simulink model "Quadrotor_Model_Roll"  (R2016a)
settings: Solver=ode45  StartTime=0.0  StopTime=20  MinStep=1e-10  RelTol=1e-1
settings Model: Creator=SRQ  LastModifiedBy=SRQ

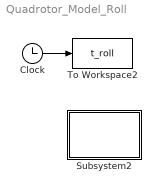
== system Quadrotor_Model_Roll ==
  Clock : Clock
  Subsystem2 : Subsystem
      mask Display: disp('翻滚通道');
  To Workspace2 : ToWorkspace  VariableName=t_roll  SampleTime=-1
  wires:
  Clock/1 -> To Workspace2/1

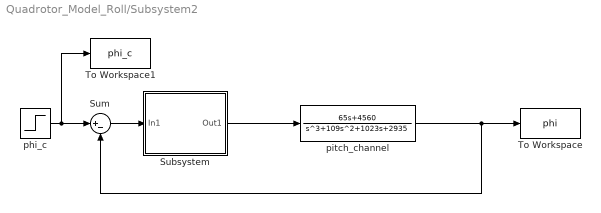
== system Quadrotor_Model_Roll/Subsystem2 ==
  Subsystem : Subsystem  mask{kp=2, ki=6, kd=0.1}
      mask Display: disp('PID');
  Sum : Sum  Inputs=|+-
  To Workspace : ToWorkspace  VariableName=phi  SampleTime=-1
  To Workspace1 : ToWorkspace  VariableName=phi_c  SampleTime=-1
  phi_c : Step  Time=0  SampleTime=0
  pitch_channel : TransferFcn  Numerator=[65 4560]  Denominator=[1 109 1023 2935]
  wires:
  phi_c/1 -> To Workspace1/1, Sum/1
  Sum/1 -> Subsystem/1(In1)
  Subsystem/1(Out1) -> pitch_channel/1
  pitch_channel/1 -> Sum/2, To Workspace/1

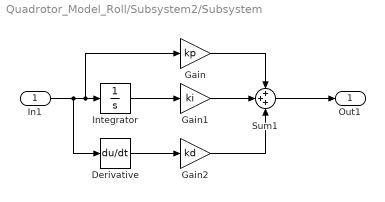
== system Quadrotor_Model_Roll/Subsystem2/Subsystem ==
  In1 : Inport
  Derivative : Derivative
  Gain : Gain  Gain=kp
  Gain1 : Gain  Gain=ki
  Gain2 : Gain  Gain=kd
  Integrator : Integrator
  Sum1 : Sum  Inputs=+++
  Out1 : Outport
  wires:
  Integrator/1 -> Gain1/1
  Derivative/1 -> Gain2/1
  Gain2/1 -> Sum1/3
  Gain/1 -> Sum1/1
  In1/1 -> Derivative/1, Gain/1, Integrator/1
  Sum1/1 -> Out1/1
  Gain1/1 -> Sum1/2
